simulink model "Universal_Bridge_2012"  (R2012b)
settings: Solver=ode45  StartTime=0.0  StopTime=0.2  RelTol=1e-3
libraries: powerlib x7, powerlib_extras x1
settings Model: Creator=Administrator  LastModifiedBy=dyj
settings DataIOCC: SignalLoggingSaveFormat=ModelDataLogs
settings OptimizationCC: ExpressionDepthLimit=128  InitFltsAndDblsToZero=on
settings DebuggingCC: SaveWithParameterizedLinksMsg=none  SignalResolutionControl=TryResolveAllWithWarning  MultiTaskDSMMsg=warning  MultiTaskCondExecSysMsg=none  FcnCallInpInsideContextMsg=EnableAllAsWarning  FrameProcessingCompatibilityMsg=error  StateNameClashWarn=none
settings CodeAppCC: CustomSymbolStrType=$N$R$M_T
settings GRTTargetCC: TargetFcnLib=ansi_tfl_tmw.mat  CodeReplacementLibrary=C89/C90 (ANSI)  GeneratePreprocessorConditionals=Use local settings  CombineOutputUpdateFcns=off  GRTInterface=on
settings SimscapeCC: SimscapeNormalizeSystem=off

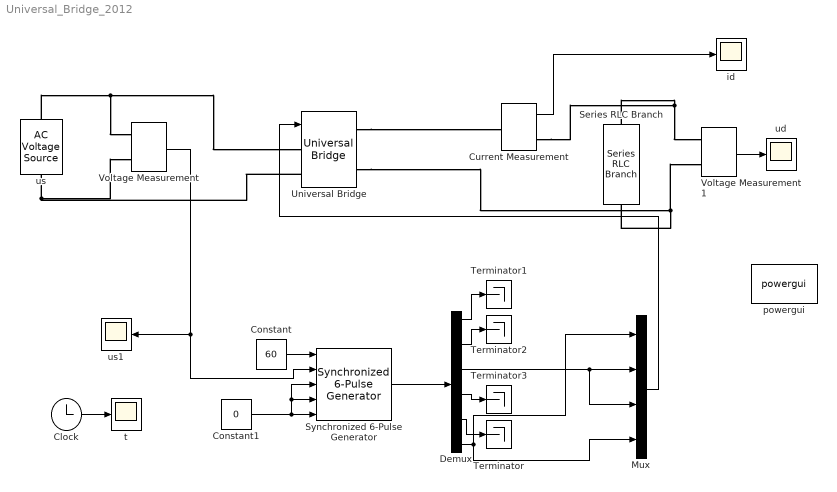
== system Universal_Bridge_2012 ==
  Clock : Clock
  Constant : Constant  Value=60
  Constant1 : Constant  Value=0
  Current Measurement : powerlib/Measurements/Current Measurement  PhasorSimulation=off  OutputType=Complex  PSBequivalent=0
  Demux : Demux  Outputs=6
  Mux : Mux
  Series RLC Branch : powerlib/Elements/Series RLC Branch  LConnTagsString=__new0  RConnTagsString=__new0  BranchType=R  Resistance=2  Inductance=10  SetiL0=off  InitialCurrent=0  Capacitance=5  Setx0=off  InitialVoltage=0  Measurements=None
  Synchronized 6-Pulse Generator : powerlib_extras/Control  Blocks/Synchronized 6-Pulse Generator  freq=60  pwidth=10  Double_Pulse=off
  Terminator{,1..3} (4 alike) : Terminator
  Universal Bridge : powerlib/Power Electronics/Universal Bridge  Arms=2  SnubberResistance=1e5  SnubberCapacitance=inf  Device=Thyristors  Ron=1e-3  Lon=0  ForwardVoltages="[  0  0  ]"  ForwardVoltage=0  GTOparameters=[ 10e-6 , 20e-6 ]  IGBTparameters=[ 1e-6 , 2e-6 ]  Measurements=None  Measurements_2=None  converterType=Rectifier
  Voltage Measurement : powerlib/Measurements/Voltage Measurement  PhasorSimulation=off  OutputType=Complex  PSBequivalent=0
  Voltage Measurement1 : powerlib/Measurements/Voltage Measurement  PhasorSimulation=off  OutputType=Complex  PSBequivalent=0
  id : Scope
      settings: TimeRange=0.4  MaxDataPoints=5000  SaveName=ScopeData  YMin=-23.71624  YMax=213.44612  SampleTime=-1
  powergui : powerlib/powergui  Priority=1  SimulationMode=Continuous  SampleTime=50e-6  frequency=60  Iterations=50  frequencyindice=50  Pbase=100e6  ErrMax=1e-4  UnitsV=kV  UnitsW=MW  buscounter=0  FunctionMessages=off  echomessages=off  EnableUseOfTLC=off  CurrentSourceSwitches=on  DisableSnubberDevices=off  DisableRonSwitches=off  DisableVfSwitches=off  DisplayEquations=off  AutomaticDiscreteSolvers=off  SolverType=Tustin/Backward Euler (TBE)  Interpol=off  ExternalGateDelay=off  methode=off  Ts=10  x0status=blocks  SPID=off  SwTol=0  HookPort=off  NonlinearTolerance=1e-4  nMaxIteration=100  ContinueOnMaxIteration=off  RestoreLinks=warning  ResistiveCurrentMeasurement=off  Frange=[0:2:500]  Ylog=off  Xlog=on  ShowGrid=off  save=off  variable=ZData  structure=0  ZoomFFT=off  StartTime=0.0  cycles=1  DisplayStyle=1  fundamental=60  FreqAxis=off  MaxFrequency=1000  frequencyindicesteady=1  RmsSteady=1  display=off
  t : Scope
      settings: TimeRange=auto  LimitDataPoints=on  MaxDataPoints=5000  SaveToWorkspace=off  SaveName=ScopeData2  YMin=-10  YMax=10  SampleTime=-1
  ud : Scope
      settings: TimeRange=0.2  LimitDataPoints=on  MaxDataPoints=5000  SaveToWorkspace=off  YMin=-47.43247  YMax=426.89225  SampleTime=-1
  us : powerlib/Electrical Sources/AC Voltage Source  Amplitude=380  Phase=0  Frequency=50  SampleTime=0  Measurements=None  BusType=swing  Pref=10e3  Qref=0  Qmin=-inf  Qmax=+inf
  us1 : Scope
      settings: TimeRange=auto  LimitDataPoints=on  MaxDataPoints=5000  SaveToWorkspace=off  SaveName=ScopeData3  YMin=-474.79905  YMax=474.79905  SampleTime=-1
  wires:
  Clock/1 -> t/1
  Voltage Measurement/1 -> Synchronized 6-Pulse Generator/2, us1/1
  Constant/1 -> Synchronized 6-Pulse Generator/1
  Constant1/1 -> Synchronized 6-Pulse Generator/3, Synchronized 6-Pulse Generator/4, Synchronized 6-Pulse Generator/5
  Synchronized 6-Pulse Generator/1 -> Demux/1
  Demux/1 -> Terminator1/1
  Demux/2 -> Terminator2/1
  Demux/4 -> Terminator3/1
  Demux/5 -> Terminator/1
  Demux/6 -> Mux/1, Mux/4
  Demux/3 -> Mux/2, Mux/3
  Mux/1 -> Universal Bridge/1
  Voltage Measurement1/1 -> ud/1
  Current Measurement/1 -> id/1
  connections:
  Universal Bridge/LConn2 -- us/LConn1 -- Voltage Measurement/LConn2
  us/RConn1 -- Universal Bridge/LConn1 -- Voltage Measurement/LConn1
  Universal Bridge/RConn1 -- Current Measurement/LConn1
  Universal Bridge/RConn2 -- Voltage Measurement1/LConn2 -- Series RLC Branch/RConn1
  Series RLC Branch/LConn1 -- Voltage Measurement1/LConn1 -- Current Measurement/RConn1
